simulink model "Tricopter_Controlled"  (R2015a)
settings: Solver=ode3  SolverMode=SingleTasking  StartTime=0.0  StopTime=inf  FixedStep=T_sim  RelTol=1e-3
values from neighbouring files (symbols this model uses):
  A_l_max_x = sqrt( (A_z_max)^2  -  g^2  )    [Run3Copter.m]
  A_l_max_y = g*tand(15)    [Run3Copter.m]
  A_z_max = Max_Thrust*3/m    [Run3Copter.m]
  Alt_0 = input(' Give the initial altitude (m): ')    [Run3Copter.m]
  B_hover_4dof = [-0.192641491537 -0.295051706147 -72.3190840892 -0.00308714144823 24.9504828653 -1.18743631629 9.87469464114e-05 6.48783896558 -0.0529805907426 -0.000387203135788 0.131620058452 2.24065603044 ... (54 elements, 6x9)]    [Effectiv_matrices.mat]
  CG_0 = [0,0,0.02]'    [SetupComplete.m]
  epsilon = 0.01    [Run3Copter.m]
  eta_23 = deg2rad(-1.3)    [Run3Copter.m]
  g = 9.81    [SetupComplete.m]
  h = 0.08    [SetupComplete.m]
  h_M = 0.064    [SetupComplete.m]
  Hover_eta_23 = deg2rad(-1.3)    [Run3Copter.m]
  Hover_throtle_1 = 0.745    [Run3Copter.m]
  Hover_throtle_23 = Hover_throtle_1/cos(Hover_eta_23)    [Run3Copter.m]
  I_BAC_0 = [ Ix,0,Ixz;0,Iy,0;Ixz,0,Iz]    [SetupComplete.m]
  Initial_Omegas = Omega_hover    [Run3Copter.m]
  Initial_Torques = Torque_hover    [Run3Copter.m]
  Ix = 0.103    [SetupComplete.m]
  Iy = 0.147    [SetupComplete.m]
  Iz = 0.237    [SetupComplete.m]
  l = 0.345    [SetupComplete.m]
  l_arm = 0.264    [SetupComplete.m]
  latitude = 52.071118    [Run3Copter.m]
  longitude = -0.627404    [Run3Copter.m]
  m = 3.51    [SetupComplete.m]
  m_0 = 2.61    [SetupComplete.m]
  m_M = 0.300    (= 0.3)    [SetupComplete.m]
  Rotation_sign = [ 1,-1,-1]    [SetupComplete.m]
  T_ctrl = 0.02    [Run3Copter.m]
  T_sim = 0.01    [Run3Copter.m]
  throtle_1 = 0*0.745    (= 0)    [Run3Copter.m]
  throtle_23 = throtle_1/cos(eta_23)    [Run3Copter.m]
  v_i0 = sqrt( 1/3*m*g/(2*rho*pi*R^2)  )    [SetupComplete.m]
undefined symbols (not defined in the file or in its folder): DOWN_0, EAST_0, Newton, NORTH_0, P_0, Q_0, R_0, Raphson, U_0, V_0, W_0
libraries: XXCopter_Control x64, simulink_extras x17, simulink x11, XXCopter x8
(part 6 of 6)

== matlab function Tricopter_Controlled/TriCopter FCS/TriCopter FCS/Control and guidance/NDI/3Copter_4_NDI&CA/Ground  model/Ground model logic and Forces and moments ==
  data: h input; F_gr_b output; mass input; q input; g parameter; Arm1 input; Arm2 input; Arm3 input
function F_gr_b    = Gorund_Forces_and_Mom( h,mass, q,g, Arm1,Arm2,Arm3)

F_gr_b=zeros(3,1);
min_h=0;

% Arm 1
Prod=HamiltonProduct([q(1);q(2);q(3);q(4)],HamiltonProduct([0;Arm1],[q(1);-q(2);-q(3);-q(4)]) ); % q . Arm .q*: From body to earth axes
h_arm1 = h + Prod(4);
% Arm 2
Prod=HamiltonProduct([q(1);q(2);q(3);q(4)],HamiltonProduct([0;Arm2],[q(1);-q(2);-q(3);-q(4)]) ); % q . Arm .q*: From body to earth axes
h_arm2 = h + Prod(4);
% Arm 3
Prod=HamiltonProduct([q(1);q(2);q(3);q(4)],HamiltonProduct([0;Arm3],[q(1);-q(2);-q(3);-q(4)]) ); % q . Arm .q*: From body to earth axes
h_arm3 = h + Prod(4);


min_h = max([h,h_arm1,h_arm2,h_arm3]);
if min_h >=-0.05 
    Prod=HamiltonProduct([q(1);-q(2);-q(3);-q(4)],HamiltonProduct([0;0;0;-mass*g],[q(1);q(2);q(3);q(4)]) ); % q* . g .q: From earth to Body axes
    F_gr_b= Prod(2:4);    
else
    F_gr_b=zeros(3,1);

end

function Product= HamiltonProduct( a,b )

Product=[ a(1)*b(1)-a(2)*b(2)-a(3)*b(3)-a(4)*b(4) ; a(1)*b(2)+a(2)*b(1)+a(3)*b(4)-a(4)*b(3)  ; a(1)*b(3)-a(2)*b(4)+a(3)*b(1)+a(4)*b(2)  ; a(1)*b(4)+a(2)*b(3)-a(3)*b(2)+a(4)*b(1) ];

== matlab function Tricopter_Controlled/TriCopter FCS/TriCopter FCS/Control and guidance/Inner PI Controller Quaternions/Limits in Ang accel/Limis eval ==
  data: Ang_Accel input size=[3,1]; Limit_up output; euler_ang input size=[3,1]; Limit_down output; l parameter; m parameter; g parameter; A_l_max_x parameter; Ix parameter; Iy parameter; Iz parameter
function [Limit_up,Limit_down]= Max_ang_accels(Ang_Accel,euler_ang,l,m,g,A_l_max_x,Ix,Iy,Iz)

Limit_up=Ang_Accel;
Limit_down=Ang_Accel;

Limit_up(1) = max(   abs( (2*m*g/3*sqrt(3)/2*l  )/Ix*cos(euler_ang(1))   ), abs(  2/3*A_l_max_x*sqrt(3)/2*l/Ix*sin(euler_ang(2)) ) )* 0.5 ;
Limit_down(1) = -Limit_up(1) ;

Limit_up(2) = max(  (l*m*g*2/3-l/2*m*g/3)/Iy*cos(euler_ang(2)) , (2*l*A_l_max_x)/Iy*sin(euler_ang(2)) )* 0.5 ;
Limit_down(2) = - max( (l/2*m*g)/Iy*cos(euler_ang(2))  , (2*l*A_l_max_x)/Iy*sin(euler_ang(2)) )* 0.5 ;


Limit_up(3) = max(  abs(  A_l_max_x*l/Iz*cos(euler_ang(1))*cos(euler_ang(2)) ) , abs(  (2*m*g/3*sqrt(3)/2*l  )/Iz*sin(euler_ang(2)) )  )* 0.5 ;
Limit_down(3) = -Limit_up(1) ;

== matlab function Tricopter_Controlled/TriCopter FCS/TriCopter FCS/Control and guidance/Inner PI Controller Quaternions/Quaternion_dot ==
  data: omega_b output; q_dot input; q input
function omega_b = Quaternion_dot(q_dot,q)

% omega_b = 2.q'*q_dot
out = 2*HamiltonProduct([q(1);- q(2:4)],q_dot);

omega_b = out(2:4);


function Product= HamiltonProduct( a,b )

Product=[ a(1)*b(1)-a(2)*b(2)-a(3)*b(3)-a(4)*b(4) ; a(1)*b(2)+a(2)*b(1)+a(3)*b(4)-a(4)*b(3)  ; a(1)*b(3)-a(2)*b(4)+a(3)*b(1)+a(4)*b(2)  ; a(1)*b(4)+a(2)*b(3)-a(3)*b(2)+a(4)*b(1) ];

== matlab function Tricopter_Controlled/TriCopter FCS/TriCopter FCS/Control and guidance/Inner PI Controller Quaternions/Get Quaternion from des euler ==
  data: phi input; q output; theta input; psi input
function q =QuaternionfromEuler(phi,theta,psi)

q=[ cos(psi/2)*cos(theta/2)*cos(phi/2)+ sin(psi/2)*sin(theta/2)*sin(phi/2) ;
      cos(psi/2)*cos(theta/2)*sin(phi/2)- sin(psi/2)*sin(theta/2)*cos(phi/2) ;
       cos(psi/2)*sin(theta/2)*cos(phi/2)+ sin(psi/2)*cos(theta/2)*sin(phi/2)   ;
        sin(psi/2)*cos(theta/2)*cos(phi/2)- cos(psi/2)*sin(theta/2)*sin(phi/2)      ]; % Esto nos da q !!!
end

== matlab function Tricopter_Controlled/TriCopter FCS/TriCopter FCS/Control and guidance/Inner PI Controller Quaternions/Attitude Controller/Build Pseudo_theta ==
  data: q input; Pseudo_theta output
function Pseudo_theta    = F_Pseudo_theta( q)


%% Actitud en Angulos de Euler y sus derivadas.
Pseudo_theta=0;
Pseudo_theta = ( 2*q(2)*q(4)-2*q(1)*q(3) ); %  pseudo-theta




end

== matlab function Tricopter_Controlled/TriCopter FCS/TriCopter FCS/Control and guidance/Inner PI Controller Quaternions/Attitude Controller/Retrieve quaternion ==
  data: Pseudoeuler_dot input size=[3,1]; q input size=[4,1]; qdot output size=[4,1]
function qdot = quat_from_Pseudoeuler(Pseudoeuler_dot, q)


%%
A = [   2/(1+( (2*q(3)*q(4)+2*q(1)*q(2))/(2*q(1)^2+2*q(4)^2-1)  )^2)*[ -(2*q(1)^2*q(2)+ 4*q(1)*q(3)*q(4)-2*q(2)*q(4)^2+q(2))  ,  q(1)*(2*q(1)^2+2*q(4)^2-1)  ,  q(4)*(2*q(1)^2+2*q(4)^2-1)  ,  -(-2*q(1)^2*q(3) +4*q(1)*q(2)*q(4)+2*q(3)*q(4)^2+q(3) ) ].* 1/(2*q(1)^2+2*q(4)^2-1)^2;...
        2*[-q(3),q(4),-q(1),q(2)];...
        2/(1+( (2*q(2)*q(3)+2*q(1)*q(4))/(2*q(1)^2+2*q(2)^2-1)  )^2)*[  -(2*q(1)^2*q(4)+4*q(1)*q(2)*q(3)-2*q(2)^2*q(4)+q(4)  ) , 1/2*(q(3)*(4*q(1)^2-4*q(2)^2-2)-8*q(1)*q(2)*q(4) )  ,  q(2)*(2*q(1)^2+2*q(2)^2-1)  , q(1)*(2*q(1)^2+2*q(2)^2-1) ].*  1/(2*q(1)^2+2*q(2)^2-1)^2 ;...
        2*[q(1),q(2),q(3),q(4)]];

qdot = pinv(A)*[Pseudoeuler_dot;0];

end

== matlab function Tricopter_Controlled/Parameters estimation/MATLAB Function ==
  data: T_yaw output; yaw input
function T_yaw = Yaw_rotate(yaw)


T_yaw=[cos(yaw),    sin(yaw),   0;
        -sin(yaw),  cos(yaw),   0;
        0,      0,              1];
